simulink model "CTS_Simulink"  (R2023a)
settings: Solver=VariableStepAuto  StartTime=0.0  StopTime=10.0  RelTol=1e-3
undefined symbols (not defined in the file): A_1, A_2, c_1, c_2, ICs, q_i0
settings Model: Creator=m260477  LastModifiedBy=m260477

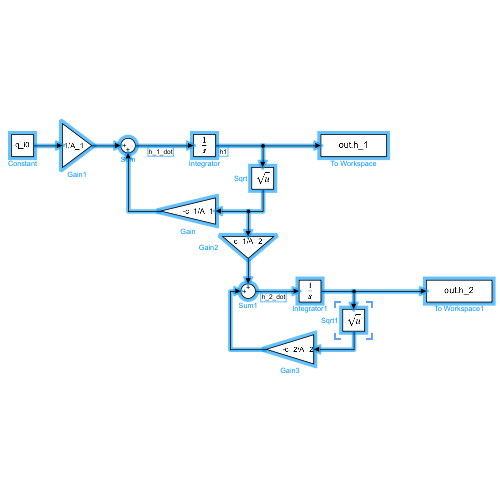
[thumbnail: Simulink's stored preview of the top-level diagram]
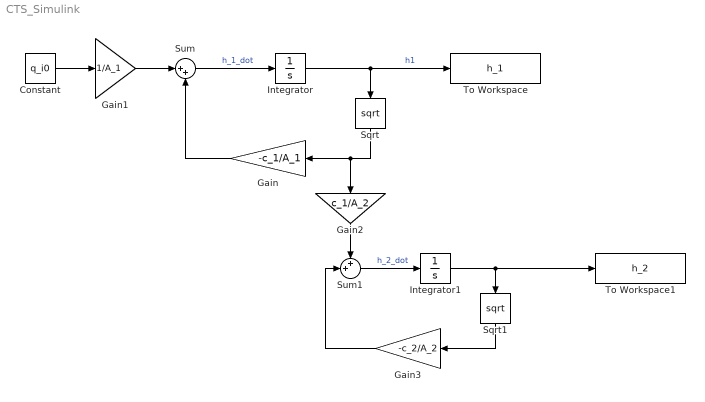
== system CTS_Simulink ==
  Constant : Constant  Value=q_i0
  Gain : Gain  Gain=-c_1/A_1
  Gain1 : Gain  Gain=1/A_1
  Gain2 : Gain  Gain=c_1/A_2
  Gain3 : Gain  Gain=-c_2/A_2
  Integrator : Integrator  InitialCondition=ICs
  Integrator1 : Integrator  InitialCondition=ICs
  Sqrt : Sqrt
  Sqrt1 : Sqrt
  Sum : Sum  Inputs=|++
  Sum1 : Sum  Inputs=++|
  To Workspace : ToWorkspace  VariableName=h_1  SaveFormat=Timeseries  SampleTime=-1
  To Workspace1 : ToWorkspace  VariableName=h_2  SaveFormat=Timeseries  SampleTime=-1
  wires:
  Integrator/1 -> To Workspace/1, Sqrt/1  "h1"
  Sqrt/1 -> Gain2/1, Gain/1
  Gain/1 -> Sum/2
  Gain1/1 -> Sum/1
  Constant/1 -> Gain1/1
  Sum/1 -> Integrator/1  "h_1_dot"
  Sum1/1 -> Integrator1/1  "h_2_dot"
  Integrator1/1 -> To Workspace1/1, Sqrt1/1
  Gain2/1 -> Sum1/1
  Sqrt1/1 -> Gain3/1
  Gain3/1 -> Sum1/2
